simulink subsystem "FuelCellElectricSystem"  (R2024a)
settings: Solver=VariableStepAuto  StartTime=0.0  StopTime=10.0  RelTol=1e-3
undefined symbols (not defined in the file): Bat, ElecThermal, Mot, PlntBattNumCellPar, PlntDCDCEff, PlntDCDCVoltInit, PlntEM1EffTbl
libraries: fl_lib x59, nesl_utility_internal x24, SimscapeFluids_lib x5, ee_lib x3, slpidlib x2, batteryecm_lib x1, simulink x1
(part 2 of 2)

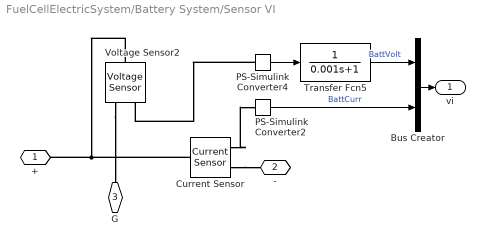
== system FuelCellElectricSystem/Battery System/Sensor VI ==
  Bus Creator : BusCreator  Inputs=2
  Current Sensor : fl_lib/Electrical/Electrical Sensors/Current Sensor
  PS-Simulink Converter2 : nesl_utility_internal/PS-Simulink Converter  PhysicalDomain=network_engine_domain  SubClassName=ps_output  LeftPortType=input  RightPortType=output  PseudoPeriodic=off  Frequencies=[]  VectorFormat=1-D array  Unit=1  AffineConversion=off
  PS-Simulink Converter4 : nesl_utility_internal/PS-Simulink Converter  PhysicalDomain=network_engine_domain  SubClassName=ps_output  LeftPortType=input  RightPortType=output  PseudoPeriodic=off  Frequencies=[]  VectorFormat=1-D array  Unit=1  AffineConversion=off
  Transfer Fcn5 : TransferFcn  Denominator=[0.001 1]
  Voltage Sensor2 : fl_lib/Electrical/Electrical Sensors/Voltage Sensor
  + : PMIOPort  Side=Left
  - : PMIOPort  Port=2  Side=Right
  G : PMIOPort  Port=3  Side=Right
  vi : Outport
  wires:
  Bus Creator/1 -> vi/1
  PS-Simulink Converter4/1 -> Transfer Fcn5/1
  PS-Simulink Converter2/1 -> Bus Creator/2  "BattCurr"
  Transfer Fcn5/1 -> Bus Creator/1  "BattVolt"
  connections:
  Current Sensor/RConn1 -- PS-Simulink Converter2/LConn1
  Voltage Sensor2/RConn2 -- G/RConn1
  Current Sensor/RConn2 -- -/RConn1
  PS-Simulink Converter4/LConn1 -- Voltage Sensor2/RConn1
  Voltage Sensor2/LConn1 -- Current Sensor/LConn1 -- +/RConn1

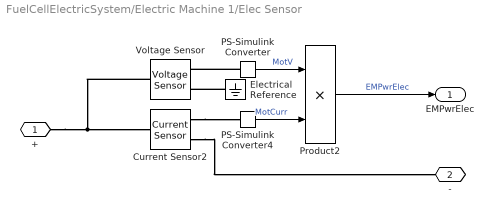
== system FuelCellElectricSystem/Electric Machine 1/Elec Sensor ==
  Current Sensor2 : fl_lib/Electrical/Electrical Sensors/Current Sensor
  Electrical Reference : fl_lib/Electrical/Electrical Elements/Electrical Reference
  PS-Simulink Converter : nesl_utility_internal/PS-Simulink Converter  PhysicalDomain=network_engine_domain  SubClassName=ps_output  LeftPortType=input  RightPortType=output  PseudoPeriodic=off  Frequencies=[]  VectorFormat=1-D array  Unit=inherit  AffineConversion=off
  PS-Simulink Converter4 : nesl_utility_internal/PS-Simulink Converter  PhysicalDomain=network_engine_domain  SubClassName=ps_output  LeftPortType=input  RightPortType=output  PseudoPeriodic=off  Frequencies=[]  VectorFormat=1-D array  Unit=1  AffineConversion=off
  Product2 : Product
  Voltage Sensor : fl_lib/Electrical/Electrical Sensors/Voltage Sensor
  + : PMIOPort  Side=Left
  - : PMIOPort  Port=2  Side=Right
  EMPwrElec : Outport
  wires:
  PS-Simulink Converter4/1 -> Product2/2  "MotCurr"
  Product2/1 -> EMPwrElec/1  "EMPwrElec"
  PS-Simulink Converter/1 -> Product2/1  "MotV"
  connections:
  Current Sensor2/RConn1 -- PS-Simulink Converter4/LConn1
  Current Sensor2/RConn2 -- -/RConn1
  +/RConn1 -- Voltage Sensor/LConn1 -- Current Sensor2/LConn1
  Electrical Reference/LConn1 -- Voltage Sensor/RConn2
  PS-Simulink Converter/LConn1 -- Voltage Sensor/RConn1

== system FuelCellElectricSystem/Electrical Cooling System/Pump Control ==
  TAmb : Inport
  TMotor : Inport  Port=2
  Add : Sum  Inputs=|-+
  PID Controller : slpidlib/PID Controller  Controller=PI  Form=Parallel  TimeDomain=Continuous-time  UseExternalTs=off  SampleTime=-1  IntegratorMethod=Forward Euler  FilterMethod=Forward Euler  ControllerParametersSource=internal  P=ElecThermal.ctrl.Kp  I=ElecThermal.ctrl.Ki  UseKiTs=off  D=0  UseExternalDerivativeSource=off  N=100  UseFilter=on  TunerSelectOption=Transfer Function Based (PID Tuner App)  ZeroCross=off  InitialConditionSource=internal  InitialConditionForIntegrator=0  InitialConditionForFilter=0  DifferentiatorICPrevScaledInput=0  ExternalReset=none  TrackingMode=off  Kt=1  LimitOutput=on  SatLimitsSource=internal  UpperSaturationLimit=0.1  LowerSaturationLimit=0  LinearizeAsGain=on  AntiWindupMode=clamping  Kb=1  LimitIntegrator=off  UpperIntegratorSaturationLimit=inf  LowerIntegratorSaturationLimit=-inf  POutMin=[]  POutMax=[]  IOutMin=[]  IOutMax=[]  DOutMin=[]  DOutMax=[]  NOutMin=[]  NOutMax=[]  SumOutMin=[]  SumOutMax=[]  SaturationOutMin=[]  SaturationOutMax=[]  PParamMin=[]  PParamMax=[]  IParamMin=[]  IParamMax=[]  DParamMin=[]  DParamMax=[]  NParamMin=[]  NParamMax=[]  KbParamMin=[]  KbParamMax=[]  KtParamMin=[]  KtParamMax=[]  KbOutMin=[]  KbOutMax=[]  KtOutMin=[]  KtOutMax=[]  IntegratorOutMin=[]  IntegratorOutMax=[]  FilterOutMin=[]  FilterOutMax=[]  SumI1OutMin=[]  SumI1OutMax=[]  SumI2OutMin=[]  SumI2OutMax=[]  SumI3OutMin=[]  SumI3OutMax=[]  SumI4OutMin=[]  SumI4OutMax=[]  SumDOutMin=[]  SumDOutMax=[]  DifferentiatorOutMin=[]  DifferentiatorOutMax=[]  FilterDiffOutCoefMin=[]  FilterDiffOutCoefMax=[]  ReciprocalOutMin=[]  ReciprocalOutMax=[]  SumDenOutMin=[]  SumDenOutMax=[]  SumNumOutMin=[]  SumNumOutMax=[]  DivideOutMin=[]  DivideOutMax=[]  UdiffTsProdOutMin=[]  UdiffTsProdOutMax=[]  NTsProdOutMin=[]  NTsProdOutMax=[]  UintegralTsProdOutMin=[]  UintegralTsProdOutMax=[]  UngainTsProdOutMin=[]  UngainTsProdOutMax=[]  ClampingZeroOutDataTypeStr=Inherit: Inherit via back propagation  ClampingZeroOutMin=[]  ClampingZeroOutMax=[]  FilterDenConstantOutDataTypeStr=Inherit: Inherit via back propagation  FilterDenConstantOutMin=[]  FilterDenConstantOutMax=[]  PCopyOutDataTypeStr=Inherit: Inherit via back propagation  PCopyOutMin=[]  PCopyOutMax=[]  NCopyOutDataTypeStr=Inherit: Inherit via back propagation  NCopyOutMin=[]  NCopyOutMax=[]  IntegratorContinuousStateAttributes=''  IntegratorStateMustResolveToSignalObject=off  IntegratorRTWStateStorageClass=Auto  FilterContinuousStateAttributes=''  FilterStateMustResolveToSignalObject=off  FilterRTWStateStorageClass=Auto  ParallelPVariant=InternalParameters  IdealPVariant=Disabled  IVariant=InternalParameters  DVariant=Disabled  IntegratorVariant=Continuous  SatVariant=Enabled  AWVariant=ContClampingParallel  PCopyVariant=Disabled  TRVariant=Disabled  FdbkBlocksVariant=Forward  IdealPFdbkVariant=Disabled  SatFdbkVariant=Disabled  DerivativeFilterVariant=Disabled  NVariant=Disabled  NCopyVariant=Disabled_SignalSpec  FilterICVariant=Disabled  IntegratorICVariant=InternalICs  ExternalResetVariant=Disabled  TRSumVariant=Passthrough  SumFdbkVariant=Disabled  SumVariant=Sum_PI  TsampFilterVariant=InternalTs  TsampNgainVariant=Passthrough  TsampIntegralVariant=Disabled_SignalSpec  ExternalSaturationOutDataTypeStr=Inherit: Same as second input  DerivativeSourceVariant=Disabled
  Sensor Dynamics : TransferFcn  Denominator=[0.1 1]
  Sensor Dynamics1 : TransferFcn  Denominator=[0.1 1]
  Pump_flw : Outport
  wires:
  TMotor/1 -> Sensor Dynamics/1
  TAmb/1 -> Sensor Dynamics1/1
  PID Controller/1 -> Pump_flw/1  "Pump_flw"
  Add/1 -> PID Controller/1
  Sensor Dynamics/1 -> Add/2
  Sensor Dynamics1/1 -> Add/1

== system FuelCellElectricSystem/Electrical Cooling System/Sensing T Amb ==
  PS-Simulink Converter1 : nesl_utility_internal/PS-Simulink Converter  PhysicalDomain=network_engine_domain  SubClassName=ps_output  LeftPortType=input  RightPortType=output  PseudoPeriodic=off  Frequencies=[]  VectorFormat=1-D array  Unit=K  AffineConversion=off
  Temperature Sensor : fl_lib/Thermal/Thermal Sensors/Temperature Sensor  temperature_measure=foundation.enum.MeasurementReference.difference
  Thermal Reference : fl_lib/Thermal/Thermal Elements/Thermal Reference
  A : PMIOPort  Side=Left
  T : Outport
  wires:
  PS-Simulink Converter1/1 -> T/1
  connections:
  Temperature Sensor/RConn1 -- Thermal Reference/LConn1
  Temperature Sensor/RConn2 -- PS-Simulink Converter1/LConn1
  Temperature Sensor/LConn1 -- A/RConn1

== system FuelCellElectricSystem/Electrical Cooling System/Sensing T Conv ==
  PS-Simulink Converter1 : nesl_utility_internal/PS-Simulink Converter  PhysicalDomain=network_engine_domain  SubClassName=ps_output  LeftPortType=input  RightPortType=output  PseudoPeriodic=off  Frequencies=[]  VectorFormat=1-D array  Unit=K  AffineConversion=off
  Temperature Sensor : fl_lib/Thermal/Thermal Sensors/Temperature Sensor  temperature_measure=foundation.enum.MeasurementReference.difference
  Thermal Reference : fl_lib/Thermal/Thermal Elements/Thermal Reference
  A : PMIOPort  Side=Left
  T : Outport
  wires:
  PS-Simulink Converter1/1 -> T/1
  connections:
  Temperature Sensor/RConn1 -- Thermal Reference/LConn1
  Temperature Sensor/RConn2 -- PS-Simulink Converter1/LConn1
  Temperature Sensor/LConn1 -- A/RConn1

== system FuelCellElectricSystem/Electrical Cooling System/Sensing T MotorR ==
  PS-Simulink Converter1 : nesl_utility_internal/PS-Simulink Converter  PhysicalDomain=network_engine_domain  SubClassName=ps_output  LeftPortType=input  RightPortType=output  PseudoPeriodic=off  Frequencies=[]  VectorFormat=1-D array  Unit=K  AffineConversion=off
  Temperature Sensor : fl_lib/Thermal/Thermal Sensors/Temperature Sensor  temperature_measure=foundation.enum.MeasurementReference.difference
  Thermal Reference : fl_lib/Thermal/Thermal Elements/Thermal Reference
  A : PMIOPort  Side=Left
  T : Outport
  wires:
  PS-Simulink Converter1/1 -> T/1
  connections:
  Temperature Sensor/LConn1 -- A/RConn1
  Temperature Sensor/RConn2 -- PS-Simulink Converter1/LConn1
  Temperature Sensor/RConn1 -- Thermal Reference/LConn1

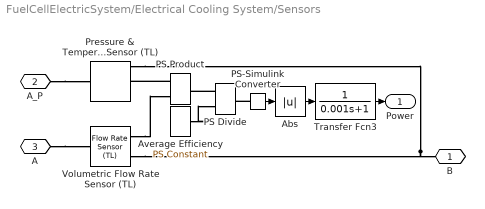
== system FuelCellElectricSystem/Electrical Cooling System/Sensors ==
  Abs : Abs  ZeroCross=off  SaturateOnIntegerOverflow=off
  Average Efficiency : fl_lib/Physical Signals/Sources/PS Constant  constant=0.9
  PS Divide : fl_lib/Physical Signals/Functions/PS Divide
  PS Product : fl_lib/Physical Signals/Functions/PS Product
  PS-Simulink Converter : nesl_utility_internal/PS-Simulink Converter  PhysicalDomain=network_engine_domain  SubClassName=ps_output  LeftPortType=input  RightPortType=output  PseudoPeriodic=off  Frequencies=[]  VectorFormat=1-D array  Unit=inherit  AffineConversion=off
  Pressure & Temperature Sensor (TL) : fl_lib/Thermal Liquid/Sensors/Pressure & Temperature Sensor (TL)  reference=foundation.enum.MeasurementReference.difference  pressure=true  pressure_spec=foundation.enum.PressureMeasementSpec.Absolute  temperature=true
      settings: InternalSimscapePortConfiguration="{\"Bottom\":[{\"id\":\"T\",\"label\":\"T\",\"type\":\"output\"}],\"Left\":[{\"id\":\"A\",\"label\":\"A\",\"type\":\"foundation.thermal_liquid.thermal_liquid\"}],\"Right\":[{\"id\":\"B\",\"label\":\"B\",\"type\":\"foundation.thermal_liquid.thermal_liquid\"},{\"id\":\"P\",\"label\":\"P\",\"type\":\"output\"}],\"Top\":[]}"
  Transfer Fcn3 : TransferFcn  Denominator=[0.001 1]
  Volumetric Flow Rate Sensor (TL) : fl_lib/Thermal Liquid/Sensors/Flow Rate Sensor (TL)  mass_flow_measure=false  volumetric_flow_measure=true  energy_flow_measure=false
      settings: InternalSimscapePortConfiguration="{\"Bottom\":[],\"Left\":[{\"id\":\"A\",\"label\":\"A\",\"type\":\"foundation.thermal_liquid.thermal_liquid\"}],\"Right\":[{\"id\":\"B\",\"label\":\"B\",\"type\":\"foundation.thermal_liquid.thermal_liquid\"},{\"id\":\"V\",\"label\":\"V\",\"type\":\"output\"}],\"Top\":[]}"
  B : PMIOPort  Side=Left
  A_P : PMIOPort  Port=2  Side=Right
  A : PMIOPort  Port=3  Side=Right
  Power : Outport
  wires:
  PS-Simulink Converter/1 -> Abs/1
  Abs/1 -> Transfer Fcn3/1
  Transfer Fcn3/1 -> Power/1
  connections:
  Pressure & Temperature Sensor (TL)/RConn1 -- Volumetric Flow Rate Sensor (TL)/RConn1 -- B/RConn1
  PS Product/LConn1 -- Pressure & Temperature Sensor (TL)/RConn2
  Volumetric Flow Rate Sensor (TL)/RConn2 -- PS Product/LConn2
  PS Divide/LConn1 -- PS Product/RConn1
  Average Efficiency/RConn1 -- PS Divide/LConn2
  PS-Simulink Converter/LConn1 -- PS Divide/RConn1
  A_P/RConn1 -- Pressure & Temperature Sensor (TL)/LConn1
  A/RConn1 -- Volumetric Flow Rate Sensor (TL)/LConn1

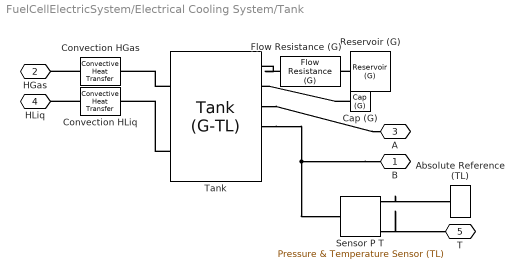
== system FuelCellElectricSystem/Electrical Cooling System/Tank ==
  Absolute Reference (TL) : fl_lib/Thermal Liquid/Elements/Absolute Reference (TL)
  Cap (G) : fl_lib/Gas/Elements/Cap (G)  p_specify=off  p_priority=None  p=0.101325 MPa  p_nominal_specify=off  p_nominal_value=1  p_nominal_unit=MPa  T_specify=off  T_priority=None  T=293.15 K  T_nominal_specify=off  T_nominal_value=1  T_nominal_unit=K
  Convection HGas : fl_lib/Thermal/Thermal Elements/Convective Heat Transfer  thermal_type=foundation.enum.constant_variable.constant  area=1e-2 m^2  heat_tr_coeff=20 W/(m^2 * K)  min_heat_tr_coeff=1e-3 W/(K*m^2)  T_specify=off  T_priority=None  T=0 K  T_nominal_specify=off  T_nominal_value=1  T_nominal_unit=K  Q_specify=off  Q_priority=None  Q=0 W  Q_nominal_specify=off  Q_nominal_value=1  Q_nominal_unit=W
  Convection HLiq : fl_lib/Thermal/Thermal Elements/Convective Heat Transfer  thermal_type=foundation.enum.constant_variable.constant  area=1e-4 m^2  heat_tr_coeff=20 W/(m^2 * K)  min_heat_tr_coeff=1e-3 W/(K*m^2)  T_specify=off  T_priority=None  T=0 K  T_nominal_specify=off  T_nominal_value=1  T_nominal_unit=K  Q_specify=off  Q_priority=None  Q=0 W  Q_nominal_specify=off  Q_nominal_value=1  Q_nominal_unit=W
  Flow Resistance (G) : fl_lib/Gas/Elements/Flow Resistance (G)  delta_p_nominal=0.001 MPa  mdot_nominal=0.1 kg/s  rho_nominal=0 kg/m^3  area=ElecThermal.Tank.areaVectorA1B1(1) m^2  laminar_fraction=1e-3
      settings: InternalSimscapePortConfiguration="{\"Bottom\":[],\"Left\":[{\"id\":\"A\",\"label\":\"A\",\"type\":\"foundation.gas.gas\"}],\"Right\":[{\"id\":\"B\",\"label\":\"B\",\"type\":\"foundation.gas.gas\"}],\"Top\":[]}"
  Reservoir (G) : fl_lib/Gas/Elements/Reservoir (G)  pressure_spec=foundation.enum.pressure_spec.atmospheric  reservoir_pressure=0.101325 MPa  reservoir_temperature=300 K  area_A=ElecThermal.Tank.areaVectorA1B1(1) m^2
  Sensor P T : fl_lib/Thermal Liquid/Sensors/Pressure & Temperature Sensor (TL)  reference=foundation.enum.MeasurementReference.difference  pressure=true  pressure_spec=foundation.enum.PressureMeasementSpec.Absolute  temperature=true
      settings: InternalSimscapePortConfiguration="{\"Bottom\":[{\"id\":\"T\",\"label\":\"T\",\"type\":\"output\"}],\"Left\":[{\"id\":\"A\",\"label\":\"A\",\"type\":\"foundation.thermal_liquid.thermal_liquid\"}],\"Right\":[{\"id\":\"B\",\"label\":\"B\",\"type\":\"foundation.thermal_liquid.thermal_liquid\"},{\"id\":\"P\",\"label\":\"P\",\"type\":\"output\"}],\"Top\":[]}"
  Tank : SimscapeFluids_lib/Thermal Liquid/Tanks & Accumulators/Tank (G-TL)  num_inlet=2  volume_total=ElecThermal.Tank.volume m^3  volume_spec=1  tank_area=ElecThermal.Tank.area m^2  level_TLU=[0, 3, 5] m  volume_TLU=[0, 4, 6] m^3  inlet_areas_A1B1=ElecThermal.Tank.areaVectorA1B1 m^2  inlet_height_A2=0.1 m  inlet_area_A2=0.01 m^2  inlet_heights_A2B2=ElecThermal.Tank.heightVector m  inlet_areas_A2B2=ElecThermal.Tank.areaVectorA2B2 m^2  inlet_heights_A2B2C2=[.1, .05, 0] m  inlet_areas_A2B2C2=[.01, .01, .01] m^2  inlet_heights_A2B2C2D2=0.1 * ones(1, 4) m  inlet_areas_A2B2C2D2=0.01 * ones(1, 4) m^2  inlet_heights_A2B2C2D2E2=0.1 * ones(1, 5) m  inlet_areas_A2B2C2D2E2=0.01 * ones(1, 5) m^2  inlet_heights_A2B2C2D2E2F2=0.1 * ones(1, 6) m  inlet_areas_A2B2C2D2E2F2=0.01 * ones(1, 6) m^2  capacity_check=0  max_liquid_capacity=ElecThermal.Tank.volume m^3  g=9.81 m/s^2  level_specify=on  level_priority=High  level=0.1 m  level_nominal_specify=off  level_nominal_value=1  level_nominal_unit=m  volume_liquid_specify=off  volume_liquid_priority=None  volume_liquid=5 m^3  volume_liquid_nominal_specify=off  volume_liquid_nominal_value=1  volume_liquid_nominal_unit=m^3  mass_liquid_specify=off  mass_liquid_priority=None  mass_liquid=5e+3 kg  mass_liquid_nominal_specify=off  mass_liquid_nominal_value=1  mass_liquid_nominal_unit=kg  T_liquid_specify=on  T_liquid_priority=High  T_liquid=300 K  T_liquid_nominal_specify=off  T_liquid_nominal_value=1  T_liquid_nominal_unit=K  p_gas_specify=off  p_gas_priority=High  p_gas=0.101325 MPa  p_gas_nominal_specify=off  p_gas_nominal_value=1  p_gas_nominal_unit=MPa  T_gas_specify=on  T_gas_priority=High  T_gas=300 K  T_gas_nominal_specify=off  T_gas_nominal_value=1  T_gas_nominal_unit=K  rho_gas_specify=off  rho_gas_priority=None  rho_gas=1.2 kg/m^3  rho_gas_nominal_specify=off  rho_gas_nominal_value=1  rho_gas_nominal_unit=kg/m^3
      settings: InternalSimscapePortConfiguration="{\"Bottom\":[],\"Left\":[{\"id\":\"A1\",\"label\":\"A1\",\"type\":\"foundation.gas.gas\"},{\"id\":\"B1\",\"label\":\"B1\",\"type\":\"foundation.gas.gas\"},{\"id\":\"A2\",\"label\":\"A2\",\"type\":\"foundation.thermal_liquid.thermal_liquid\"},{\"id\":\"B2\",\"label\":\"B2\",\"type\":\"foundation.thermal_liquid.thermal_liquid\"}],\"Right\":[{\"id\":\"H1\",\"label\":\"H1\",\"type\":\"foundation.thermal.thermal\"},{\"id\":\"H2\",\"label\":\"H2\",\"type\":\"foundation.thermal.thermal\"}],\"Top\":[{\"id\":\"V_out\",\"label\":\"V\",\"type\":\"output\"},{\"id\":\"L_out\",\"label\":\"L\",\"type\":\"output\"}]}"
  B : PMIOPort  Side=Left
  HGas : PMIOPort  Port=2  Side=Left
  A : PMIOPort  Port=3  Side=Right
  HLiq : PMIOPort  Port=4  Side=Left
  T : PMIOPort  Port=5  Side=Right
  connections:
  Tank/RConn1 -- Convection HGas/LConn1
  Convection HLiq/RConn1 -- HLiq/RConn1
  Sensor P T/RConn3 -- T/RConn1
  Sensor P T/RConn1 -- Absolute Reference (TL)/LConn1
  B/RConn1 -- Sensor P T/LConn1 -- Tank/LConn4
  Cap (G)/LConn1 -- Tank/LConn2
  Convection HGas/RConn1 -- HGas/RConn1
  Reservoir (G)/LConn1 -- Flow Resistance (G)/LConn1
  Tank/RConn2 -- Convection HLiq/LConn1
  Tank/LConn3 -- A/RConn1
  Flow Resistance (G)/RConn1 -- Tank/LConn1

== system FuelCellElectricSystem/Electrical Cooling System/Thermal Circuit Converter FC ==
  Conductive Heat Transfer : fl_lib/Thermal/Thermal Elements/Conductive Heat Transfer  thermal_type=foundation.enum.ConstantVariableTabulated.Constant  wall_geometry=foundation.enum.ConductionWallGeometry.Planar  area=0.01*pi*1 m^2  thickness=0.004 m  d_in=0.05 m  d_out=0.1 m  L=1 m  th_cond_min=10 W/(K*m)  th_cond="237;  %Al W/(m*K)"  th_cond_TLU=[413, 401, 392, 383, 371, 357, 342] W/(K*m)  temp_TLU=[200, 273, 400, 600, 800, 1000, 1200] K  T_specify=off  T_priority=None  T=0 K  T_nominal_specify=off  T_nominal_value=1  T_nominal_unit=K  Q_specify=off  Q_priority=None  Q=0 W  Q_nominal_specify=off  Q_nominal_value=1  Q_nominal_unit=W
  Thermal Mass : fl_lib/Thermal/Thermal Elements/Thermal Mass  mass_type=foundation.enum.constant_variable.constant  mass=ElecThermal.TM1.mass kg  sp_heat=ElecThermal.TM1.sh J/kg/K  mass_min=1e-6 kg  num_ports=foundation.enum.numPorts2.one  m_specify=off  m_priority=High  m=1 kg  m_nominal_specify=off  m_nominal_value=1  m_nominal_unit=kg  T_specify=off  T_priority=High  T=300 K  T_nominal_specify=off  T_nominal_value=1  T_nominal_unit=K  Q_specify=off  Q_priority=None  Q=0 W  Q_nominal_specify=off  Q_nominal_value=1  Q_nominal_unit=W
  A : PMIOPort  Side=Left
  B : PMIOPort  Port=2  Side=Right
  connections:
  Conductive Heat Transfer/LConn1 -- A/RConn1
  B/RConn1 -- Thermal Mass/LConn1 -- Conductive Heat Transfer/RConn1

== system FuelCellElectricSystem/Electrical Cooling System/Thermal Circuit Motor ==
  Case-Ambient Insulated : fl_lib/Thermal/Thermal Elements/Perfect Insulator  T_specify=off  T_priority=None  T=0 K  T_nominal_specify=off  T_nominal_value=1  T_nominal_unit=K
  Iron Stack-Case Conductance : fl_lib/Thermal/Thermal Elements/Conductive Heat Transfer  thermal_type=foundation.enum.ConstantVariableTabulated.Constant  wall_geometry=foundation.enum.ConductionWallGeometry.Planar  area=Mot.ironStack.area cm^2  thickness=Mot.ironStack.thick cm  d_in=0.05 m  d_out=0.1 m  L=1 m  th_cond_min=10 W/(K*m)  th_cond=Mot.ironStack.cond W/(m*K)  th_cond_TLU=[413, 401, 392, 383, 371, 357, 342] W/(K*m)  temp_TLU=[200, 273, 400, 600, 800, 1000, 1200] K  T_specify=off  T_priority=None  T=0 K  T_nominal_specify=off  T_nominal_value=1  T_nominal_unit=K  Q_specify=off  Q_priority=None  Q=0 W  Q_nominal_specify=off  Q_nominal_value=1  Q_nominal_unit=W
  Motor Case Thermal Mass : fl_lib/Thermal/Thermal Elements/Thermal Mass  mass_type=foundation.enum.constant_variable.constant  mass=Mot.ironStack.mass kg  sp_heat=Mot.ironStack.sh J/kg/K  mass_min=1e-6 kg  num_ports=foundation.enum.numPorts2.one  m_specify=off  m_priority=High  m=1 kg  m_nominal_specify=off  m_nominal_value=1  m_nominal_unit=kg  T_specify=off  T_priority=High  T=300 K  T_nominal_specify=off  T_nominal_value=1  T_nominal_unit=K  Q_specify=off  Q_priority=None  Q=0 W  Q_nominal_specify=off  Q_nominal_value=1  Q_nominal_unit=W
  Stator Iron Thermal Mass : fl_lib/Thermal/Thermal Elements/Thermal Mass  mass_type=foundation.enum.constant_variable.constant  mass=Mot.windingIron.mass kg  sp_heat=Mot.windingIron.sh J/kg/K  mass_min=1e-6 kg  num_ports=foundation.enum.numPorts2.one  m_specify=off  m_priority=High  m=1 kg  m_nominal_specify=off  m_nominal_value=1  m_nominal_unit=kg  T_specify=off  T_priority=High  T=300 K  T_nominal_specify=off  T_nominal_value=1  T_nominal_unit=K  Q_specify=off  Q_priority=None  Q=0 W  Q_nominal_specify=off  Q_nominal_value=1  Q_nominal_unit=W
  Winding Conductance : fl_lib/Thermal/Thermal Elements/Conductive Heat Transfer  thermal_type=foundation.enum.ConstantVariableTabulated.Constant  wall_geometry=foundation.enum.ConductionWallGeometry.Planar  area=Mot.winding.area cm^2  thickness=Mot.winding.thick cm  d_in=0.05 m  d_out=0.1 m  L=1 m  th_cond_min=10 W/(K*m)  th_cond=Mot.winding.cond W/(m*K)  th_cond_TLU=[413, 401, 392, 383, 371, 357, 342] W/(K*m)  temp_TLU=[200, 273, 400, 600, 800, 1000, 1200] K  T_specify=off  T_priority=None  T=0 K  T_nominal_specify=off  T_nominal_value=1  T_nominal_unit=K  Q_specify=off  Q_priority=None  Q=0 W  Q_nominal_specify=off  Q_nominal_value=1  Q_nominal_unit=W
  Winding Thermal Mass : fl_lib/Thermal/Thermal Elements/Thermal Mass  mass_type=foundation.enum.constant_variable.constant  mass=Mot.winding.mass kg  sp_heat=Mot.winding.sh J/kg/K  mass_min=1e-6 kg  num_ports=foundation.enum.numPorts2.one  m_specify=off  m_priority=High  m=1 kg  m_nominal_specify=off  m_nominal_value=1  m_nominal_unit=kg  T_specify=off  T_priority=High  T=300 K  T_nominal_specify=off  T_nominal_value=1  T_nominal_unit=K  Q_specify=off  Q_priority=None  Q=0 W  Q_nominal_specify=off  Q_nominal_value=1  Q_nominal_unit=W
  Winding-Iron Conductance : fl_lib/Thermal/Thermal Elements/Conductive Heat Transfer  thermal_type=foundation.enum.ConstantVariableTabulated.Constant  wall_geometry=foundation.enum.ConductionWallGeometry.Planar  area=Mot.windingIron.area cm^2  thickness=Mot.windingIron.thick cm  d_in=0.05 m  d_out=0.1 m  L=1 m  th_cond_min=10 W/(K*m)  th_cond=Mot.windingIron.cond W/(m*K)  th_cond_TLU=[413, 401, 392, 383, 371, 357, 342] W/(K*m)  temp_TLU=[200, 273, 400, 600, 800, 1000, 1200] K  T_specify=off  T_priority=None  T=0 K  T_nominal_specify=off  T_nominal_value=1  T_nominal_unit=K  Q_specify=off  Q_priority=None  Q=0 W  Q_nominal_specify=off  Q_nominal_value=1  Q_nominal_unit=W
  A : PMIOPort  Side=Left
  B : PMIOPort  Port=2  Side=Right
  connections:
  Winding Conductance/LConn1 -- Winding-Iron Conductance/RConn1 -- Winding Thermal Mass/LConn1
  Motor Case Thermal Mass/LConn1 -- Iron Stack-Case Conductance/RConn1 -- Case-Ambient Insulated/LConn1
  Stator Iron Thermal Mass/LConn1 -- Iron Stack-Case Conductance/LConn1 -- Winding-Iron Conductance/LConn1 -- B/RConn1
  Winding Conductance/RConn1 -- A/RConn1

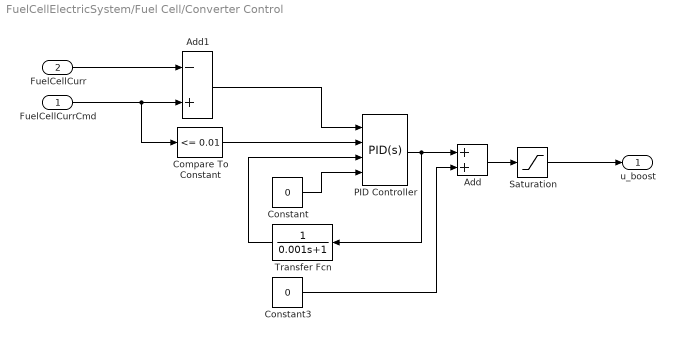
== system FuelCellElectricSystem/Fuel Cell/Converter Control ==
  FuelCellCurrCmd : Inport
  FuelCellCurr : Inport  Port=2
  Add : Sum
  Add1 : Sum  Inputs=-+
  Compare To Constant : simulink/Logic and Bit Operations/Compare To Constant  relop=<=  const=0.01  OutDataTypeStr=boolean  ZeroCross=off
  Constant : Constant  Value=0  SampleTime=-1
  Constant3 : Constant  Value=0  SampleTime=-1
  PID Controller : slpidlib/PID Controller  Controller=PID  Form=Parallel  TimeDomain=Continuous-time  UseExternalTs=off  SampleTime=-1  IntegratorMethod=Forward Euler  FilterMethod=Forward Euler  ControllerParametersSource=internal  P=0.006  I=0.01  UseKiTs=off  D=0  UseExternalDerivativeSource=off  N=100  UseFilter=on  TunerSelectOption=Transfer Function Based (PID Tuner App)  InitialConditionSource=external  InitialConditionForIntegrator=0  InitialConditionForFilter=0  DifferentiatorICPrevScaledInput=0  ExternalReset=falling  TrackingMode=off  Kt=1  LimitOutput=on  SatLimitsSource=internal  UpperSaturationLimit=1  LowerSaturationLimit=-1  LinearizeAsGain=on  AntiWindupMode=none  Kb=1  LimitIntegrator=off  UpperIntegratorSaturationLimit=inf  LowerIntegratorSaturationLimit=-inf  POutMin=[]  POutMax=[]  IOutMin=[]  IOutMax=[]  DOutMin=[]  DOutMax=[]  NOutMin=[]  NOutMax=[]  SumOutMin=[]  SumOutMax=[]  SaturationOutMin=[]  SaturationOutMax=[]  PParamMin=[]  PParamMax=[]  IParamMin=[]  IParamMax=[]  DParamMin=[]  DParamMax=[]  NParamMin=[]  NParamMax=[]  KbParamMin=[]  KbParamMax=[]  KtParamMin=[]  KtParamMax=[]  KbOutMin=[]  KbOutMax=[]  KtOutMin=[]  KtOutMax=[]  IntegratorOutMin=[]  IntegratorOutMax=[]  FilterOutMin=[]  FilterOutMax=[]  SumI1OutMin=[]  SumI1OutMax=[]  SumI2OutMin=[]  SumI2OutMax=[]  SumI3OutMin=[]  SumI3OutMax=[]  SumI4OutMin=[]  SumI4OutMax=[]  SumDOutMin=[]  SumDOutMax=[]  DifferentiatorOutMin=[]  DifferentiatorOutMax=[]  FilterDiffOutCoefMin=[]  FilterDiffOutCoefMax=[]  ReciprocalOutMin=[]  ReciprocalOutMax=[]  SumDenOutMin=[]  SumDenOutMax=[]  SumNumOutMin=[]  SumNumOutMax=[]  DivideOutMin=[]  DivideOutMax=[]  UdiffTsProdOutMin=[]  UdiffTsProdOutMax=[]  NTsProdOutMin=[]  NTsProdOutMax=[]  UintegralTsProdOutMin=[]  UintegralTsProdOutMax=[]  UngainTsProdOutMin=[]  UngainTsProdOutMax=[]  ClampingZeroOutDataTypeStr=Inherit: Inherit via back propagation  ClampingZeroOutMin=[]  ClampingZeroOutMax=[]  FilterDenConstantOutDataTypeStr=Inherit: Inherit via back propagation  FilterDenConstantOutMin=[]  FilterDenConstantOutMax=[]  PCopyOutDataTypeStr=Inherit: Inherit via back propagation  PCopyOutMin=[]  PCopyOutMax=[]  NCopyOutDataTypeStr=Inherit: Inherit via back propagation  NCopyOutMin=[]  NCopyOutMax=[]  IntegratorContinuousStateAttributes=''  IntegratorStateMustResolveToSignalObject=off  IntegratorRTWStateStorageClass=Auto  FilterContinuousStateAttributes=''  FilterStateMustResolveToSignalObject=off  FilterRTWStateStorageClass=Auto  ParallelPVariant=InternalParameters  IdealPVariant=Disabled  IVariant=InternalParameters  DVariant=InternalParameters  IntegratorVariant=Continuous  SatVariant=Enabled  AWVariant=Passthrough  PCopyVariant=Disabled  TRVariant=Disabled  FdbkBlocksVariant=Forward  IdealPFdbkVariant=Disabled  SatFdbkVariant=Disabled  DerivativeFilterVariant=ContFilter  NVariant=InternalParameters  NCopyVariant=Disabled  FilterICVariant=ExternalICs  IntegratorICVariant=ExternalICs  ExternalResetVariant=ExternalReset  TRSumVariant=Passthrough  SumFdbkVariant=Disabled  SumVariant=Sum_PID  TsampFilterVariant=InternalTs  TsampNgainVariant=Passthrough  TsampIntegralVariant=Disabled_SignalSpec  ExternalSaturationOutDataTypeStr=Inherit: Same as second input  DerivativeSourceVariant=ErrorSignal
  Saturation : Saturate  UpperLimit=1  LowerLimit=0  ZeroCross=off
  Transfer Fcn : TransferFcn  Denominator=[0.001 1]
  u_boost : Outport
  wires:
  Constant3/1 -> Add/2
  PID Controller/1 -> Add/1, Transfer Fcn/1
  FuelCellCurr/1 -> Add1/1
  Add/1 -> Saturation/1
  FuelCellCurrCmd/1 -> Compare To Constant/1, Add1/2
  Add1/1 -> PID Controller/1
  Transfer Fcn/1 -> PID Controller/3
  Constant/1 -> PID Controller/4
  Compare To Constant/1 -> PID Controller/2
  Saturation/1 -> u_boost/1

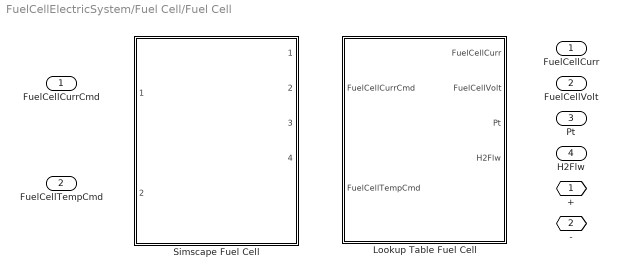
== system FuelCellElectricSystem/Fuel Cell/Fuel Cell ==
  FuelCellCurrCmd : Inport
  FuelCellTempCmd : Inport  Port=2
  Lookup Table Fuel Cell : Subsystem  VariantControl=1
      settings: PortSchema="{\"entries\":[{\"content\":{\"sides\":[{\"content\":{\"connectorIds\":[]},\"type\":\"ConnectorPlacement.EquallySpacedRectSide\",\"uuid\":\"32248e1c-8adb-4301-a735-652c844f38d9\"},{\"content\":{\"connectorIds\":[],\"side\":\"RIGHT\"},\"type\":\"ConnectorPlacement.EquallySpacedRectSide\",\"uuid\":\"e199895e-2a46-4791-8ec6-c72fbddb281a\"},{\"content\":{\"connectorIds\":[\"In1\",\"In2\"],\"side\":\"TOP\"},\"type\":\"ConnectorPlacement.EquallySpacedRectSide\",\"uuid\":\"d27f5cfc-8d50-4a08-b63d-60966cdd3a3e\"},{\"content\":{\"connectorIds\":[\"Out1\",\"Out2\",\"Out3\",\"Out4\",\"RConn1\",\"RConn2\"],\"side\":\"BOTTOM\"},\"type\":\"ConnectorPlacement.EquallySpacedRectSide\",\"uuid\":\"4de9f516-5cfd-4c93-92a2-161937995774\"}]},\"type\":\"ConnectorPlacement.EquallySpacedConnector\",\"uuid\":\"ebb74780-6fd4-4e24-9636-290cc1e1e603\"}],\"packageUris\":[\"http://schema.mathworks.com/mf0/Connector/R2020b\"],\"version\":\"1.0\"}"
  Simscape Fuel Cell : Subsystem  VariantControl=Choice_1  ReferencedSubsystem=FuelCellCore
  + : PMIOPort  Side=Right
  - : PMIOPort  Port=2  Side=Right
  FuelCellCurr : Outport
  FuelCellVolt : Outport  Port=2
  Pt : Outport  Port=3
  H2Flw : Outport  Port=4

== system FuelCellElectricSystem/Fuel Cell/Thermal1 ==
  Controlled Heat Flow Rate Source : fl_lib/Thermal/Thermal Sources/Controlled Heat Flow Rate Source
  PS Gain : fl_lib/Physical Signals/Functions/PS Gain  gain=0.001 Ohm
  PS Math Function : fl_lib/Physical Signals/Functions/PS Math Function  fcn_choice=foundation.enum.math_function.square  v=1
  Thermal Mass : fl_lib/Thermal/Thermal Elements/Thermal Mass  mass_type=foundation.enum.constant_variable.constant  mass=500 kg  sp_heat=447 J/kg/K  mass_min=1e-6 kg  num_ports=foundation.enum.numPorts2.one  m_specify=off  m_priority=High  m=1 kg  m_nominal_specify=off  m_nominal_value=1  m_nominal_unit=kg  T_specify=off  T_priority=High  T=300 K  T_nominal_specify=off  T_nominal_value=1  T_nominal_unit=K  Q_specify=off  Q_priority=None  Q=0 W  Q_nominal_specify=off  Q_nominal_value=1  Q_nominal_unit=W
  Thermal Reference2 : fl_lib/Thermal/Thermal Elements/Thermal Reference
  H : PMIOPort  Side=Right
  i : PMIOPort  Port=2  Side=Left
  connections:
  H/RConn1 -- Controlled Heat Flow Rate Source/LConn1 -- Thermal Mass/LConn1
  i/RConn1 -- PS Math Function/LConn1
  Thermal Reference2/LConn1 -- Controlled Heat Flow Rate Source/RConn2
  PS Math Function/RConn1 -- PS Gain/LConn1
  Controlled Heat Flow Rate Source/RConn1 -- PS Gain/RConn1

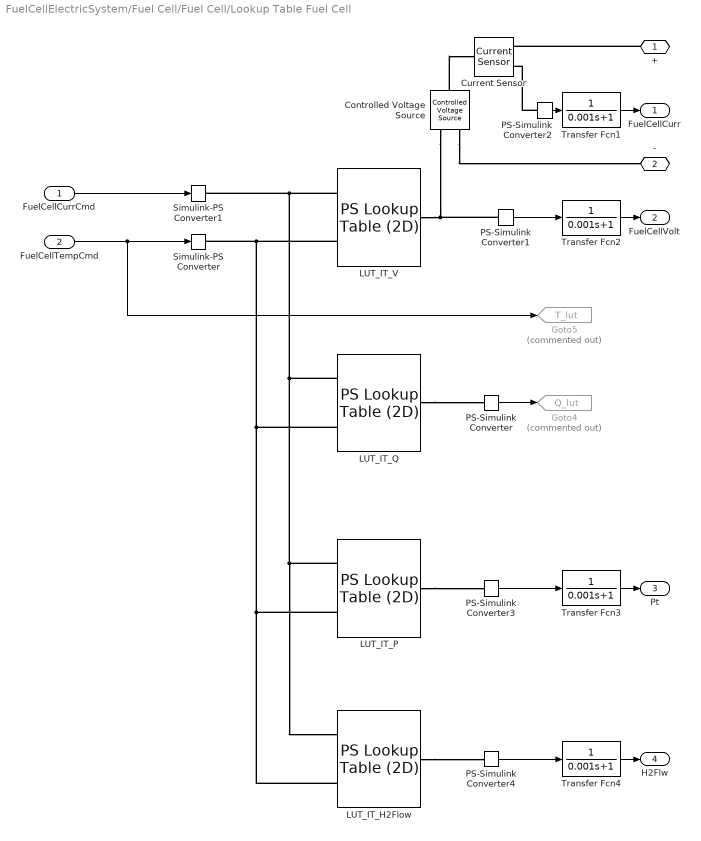
== system FuelCellElectricSystem/Fuel Cell/Fuel Cell/Lookup Table Fuel Cell ==
  FuelCellCurrCmd : Inport
  FuelCellTempCmd : Inport  Port=2
  Controlled Voltage Source : fl_lib/Electrical/Electrical Sources/Controlled Voltage Source
  Current Sensor : fl_lib/Electrical/Electrical Sensors/Current Sensor
  Goto4 : Goto  Commented=on  GotoTag=Q_lut  TagVisibility=global
  Goto5 : Goto  Commented=on  GotoTag=T_lut  TagVisibility=global
  LUT_IT_H2Flow : fl_lib/Physical Signals/Lookup Tables/PS Lookup Table (2D)  x1=f_fc_currcmd_bpt A  x2=f_fc_tmpcmd_bpt  f=f_fc_h2flow kg/s  interp_method=simscape.enum.interpolation.linear  extrap_method=simscape.enum.extrapolation.linear
      settings: AttributesFormatString=%<f>
  LUT_IT_P : fl_lib/Physical Signals/Lookup Tables/PS Lookup Table (2D)  x1=f_fc_currcmd_bpt A  x2=f_fc_tmpcmd_bpt  f=f_fc_auxpower W  interp_method=simscape.enum.interpolation.linear  extrap_method=simscape.enum.extrapolation.linear
      settings: AttributesFormatString=%<f>
  LUT_IT_Q : fl_lib/Physical Signals/Lookup Tables/PS Lookup Table (2D)  x1=f_fc_currcmd_bpt A  x2=f_fc_tmpcmd_bpt  f=f_fc_heatflow W  interp_method=simscape.enum.interpolation.linear  extrap_method=simscape.enum.extrapolation.linear
      settings: AttributesFormatString=%<f>
  LUT_IT_V : fl_lib/Physical Signals/Lookup Tables/PS Lookup Table (2D)  x1=f_fc_currcmd_bpt A  x2=f_fc_tmpcmd_bpt  f=f_fc_voltage V  interp_method=simscape.enum.interpolation.linear  extrap_method=simscape.enum.extrapolation.linear
      settings: AttributesFormatString=%<f>
  PS-Simulink Converter : nesl_utility_internal/PS-Simulink Converter  PhysicalDomain=network_engine_domain  SubClassName=ps_output  LeftPortType=input  RightPortType=output  PseudoPeriodic=off  Frequencies=[]  VectorFormat=1-D array  Unit=kW  AffineConversion=off
  PS-Simulink Converter1 : nesl_utility_internal/PS-Simulink Converter  PhysicalDomain=network_engine_domain  SubClassName=ps_output  LeftPortType=input  RightPortType=output  PseudoPeriodic=off  Frequencies=[]  VectorFormat=1-D array  Unit=inherit  AffineConversion=off
  PS-Simulink Converter2 : nesl_utility_internal/PS-Simulink Converter  PhysicalDomain=network_engine_domain  SubClassName=ps_output  LeftPortType=input  RightPortType=output  PseudoPeriodic=off  Frequencies=[]  VectorFormat=1-D array  Unit=1  AffineConversion=off
  PS-Simulink Converter3 : nesl_utility_internal/PS-Simulink Converter  PhysicalDomain=network_engine_domain  SubClassName=ps_output  LeftPortType=input  RightPortType=output  PseudoPeriodic=off  Frequencies=[]  VectorFormat=1-D array  Unit=W  AffineConversion=off
  PS-Simulink Converter4 : nesl_utility_internal/PS-Simulink Converter  PhysicalDomain=network_engine_domain  SubClassName=ps_output  LeftPortType=input  RightPortType=output  PseudoPeriodic=off  Frequencies=[]  VectorFormat=1-D array  Unit=kg/s  AffineConversion=off
  Simulink-PS Converter : nesl_utility_internal/Simulink-PS Converter  PhysicalDomain=network_engine_domain  SubClassName=ps_input  LeftPortType=input  RightPortType=output  PseudoPeriodic=off  Frequencies=[]  NoiseDistribution=none  NoiseParameters=[]  Unit=1  AffineConversion=off  FilteringAndDerivatives=provide  SimscapeFilterOrder=1  InputFilterTimeConstant=0.001  UdotUserProvided=0
  Simulink-PS Converter1 : nesl_utility_internal/Simulink-PS Converter  PhysicalDomain=network_engine_domain  SubClassName=ps_input  LeftPortType=input  RightPortType=output  PseudoPeriodic=off  Frequencies=[]  NoiseDistribution=none  NoiseParameters=[]  Unit=A  AffineConversion=off  FilteringAndDerivatives=provide  SimscapeFilterOrder=1  InputFilterTimeConstant=0.001  UdotUserProvided=0
  Transfer Fcn{1..4} (4 alike) : TransferFcn  Denominator=[0.001 1]
  + : PMIOPort  Side=Right
  - : PMIOPort  Port=2  Side=Right
  FuelCellCurr : Outport
  FuelCellVolt : Outport  Port=2
  Pt : Outport  Port=3
  H2Flw : Outport  Port=4
  wires:
  FuelCellTempCmd/1 -> Goto5/1, Simulink-PS Converter/1
  PS-Simulink Converter/1 -> Goto4/1
  FuelCellCurrCmd/1 -> Simulink-PS Converter1/1
  PS-Simulink Converter2/1 -> Transfer Fcn1/1
  PS-Simulink Converter1/1 -> Transfer Fcn2/1
  Transfer Fcn1/1 -> FuelCellCurr/1
  Transfer Fcn2/1 -> FuelCellVolt/1
  PS-Simulink Converter3/1 -> Transfer Fcn3/1
  Transfer Fcn3/1 -> Pt/1
  Transfer Fcn4/1 -> H2Flw/1
  PS-Simulink Converter4/1 -> Transfer Fcn4/1
  connections:
  Simulink-PS Converter/RConn1 -- LUT_IT_H2Flow/LConn2 -- LUT_IT_P/LConn2 -- LUT_IT_Q/LConn2 -- LUT_IT_V/LConn2
  Controlled Voltage Source/LConn1 -- Current Sensor/LConn1
  Controlled Voltage Source/RConn1 -- LUT_IT_V/RConn1 -- PS-Simulink Converter1/LConn1
  Simulink-PS Converter1/RConn1 -- LUT_IT_P/LConn1 -- LUT_IT_H2Flow/LConn1 -- LUT_IT_Q/LConn1 -- LUT_IT_V/LConn1
  LUT_IT_Q/RConn1 -- PS-Simulink Converter/LConn1
  PS-Simulink Converter2/LConn1 -- Current Sensor/RConn1
  Controlled Voltage Source/RConn2 -- -/RConn1
  +/RConn1 -- Current Sensor/RConn2
  LUT_IT_P/RConn1 -- PS-Simulink Converter3/LConn1
  LUT_IT_H2Flow/RConn1 -- PS-Simulink Converter4/LConn1
